simulink model "silnik elektryczny"  (R2025b)
settings: Solver=ode4  StartTime=0.0  StopTime=5  FixedStep=0.001  RelTol=1e-3
InitFcn:
  | Jzr = 0.027
  | Uamax = 220
  | Ra = 0.8
  | La = 0.1
  | Rf = 0.65
  | Lf = 0.1
  | Mo = 50
  | fobc = 13
  | k = 0.05
libraries: slpidlib x1, simulink x1
settings Model: Creator=maciuś  LastModifiedBy=maciuś

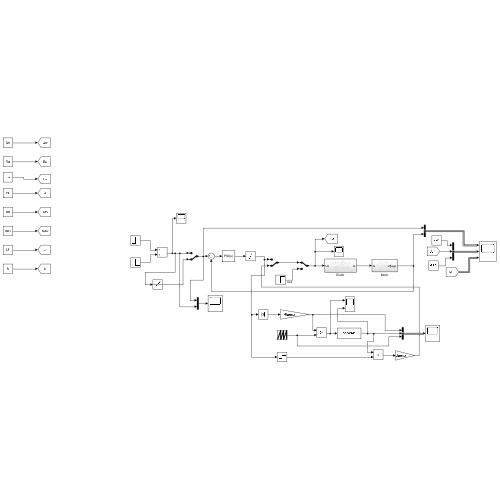
[thumbnail: Simulink's stored preview of the top-level diagram]
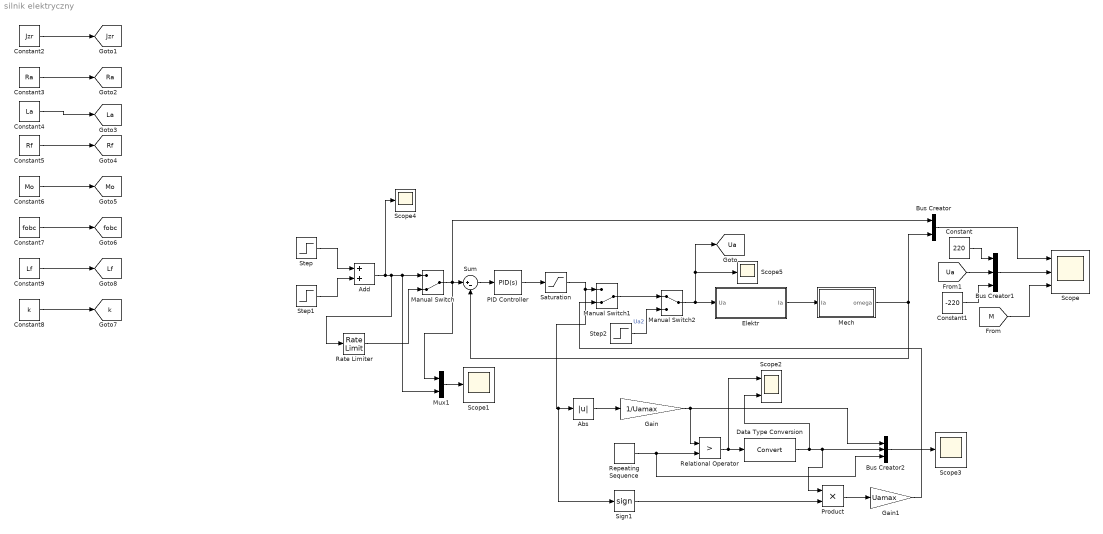
== system silnik elektryczny ==
  Abs : Abs  SaturateOnIntegerOverflow=off
  Add : Sum
  Bus Creator : BusCreator  Inputs=2
  Bus Creator1 : BusCreator  Inputs=3
  Bus Creator2 : BusCreator  Inputs=3
  Constant : Constant  Value=220
  Constant1 : Constant  Value=-220
  Constant2 : Constant  Value=Jzr
  Constant3 : Constant  Value=Ra
  Constant4 : Constant  Value=La
  Constant5 : Constant  Value=Rf
  Constant6 : Constant  Value=Mo
  Constant7 : Constant  Value=fobc
  Constant8 : Constant  Value=k
  Constant9 : Constant  Value=Lf
  Data Type Conversion : DataTypeConversion  SaturateOnIntegerOverflow=off  RndMeth=Floor
  Elektr : Subsystem
  Gain : Gain  Gain=1/Uamax
  Gain1 : Gain  Gain=Uamax
  Manual Switch : ManualSwitch  CurrentSetting=0
  Manual Switch1 : ManualSwitch  CurrentSetting=0
  Manual Switch2 : ManualSwitch
  Mech : Subsystem
  Mux1 : Mux  Inputs=2
  PID Controller : slpidlib/PID Controller  Controller=PID  Form=Ideal  TimeDomain=Continuous-time  UseExternalTs=off  SampleTime=-1  IntegratorMethod=Forward Euler  FilterMethod=Forward Euler  ControllerParametersSource=internal  P=8  I=5  UseKiTs=off  D=0.07  UseExternalDerivativeSource=off  N=100  UseFilter=on  TunerSelectOption=Transfer Function Based (PID Tuner App)  InitialConditionSource=internal  InitialConditionForIntegrator=0  InitialConditionForFilter=0  DifferentiatorICPrevScaledInput=0  ExternalReset=none  TrackingMode=off  Kt=1  LimitOutput=off  SatLimitsSource=internal  UpperSaturationLimit=inf  LowerSaturationLimit=-inf  LinearizeAsGain=on  AntiWindupMode=none  Kb=1  LimitIntegrator=off  UpperIntegratorSaturationLimit=inf  LowerIntegratorSaturationLimit=-inf  POutMin=[]  POutMax=[]  IOutMin=[]  IOutMax=[]  DOutMin=[]  DOutMax=[]  NOutMin=[]  NOutMax=[]  SumOutMin=[]  SumOutMax=[]  SaturationOutMin=[]  SaturationOutMax=[]  PParamMin=[]  PParamMax=[]  IParamMin=[]  IParamMax=[]  DParamMin=[]  DParamMax=[]  NParamMin=[]  NParamMax=[]  KbParamMin=[]  KbParamMax=[]  KtParamMin=[]  KtParamMax=[]  KbOutMin=[]  KbOutMax=[]  KtOutMin=[]  KtOutMax=[]  IntegratorOutMin=[]  IntegratorOutMax=[]  FilterOutMin=[]  FilterOutMax=[]  SumI1OutMin=[]  SumI1OutMax=[]  SumI2OutMin=[]  SumI2OutMax=[]  SumI3OutMin=[]  SumI3OutMax=[]  SumI4OutMin=[]  SumI4OutMax=[]  SumDOutMin=[]  SumDOutMax=[]  DifferentiatorOutMin=[]  DifferentiatorOutMax=[]  FilterDiffOutCoefMin=[]  FilterDiffOutCoefMax=[]  ReciprocalOutMin=[]  ReciprocalOutMax=[]  SumDenOutMin=[]  SumDenOutMax=[]  SumNumOutMin=[]  SumNumOutMax=[]  DivideOutMin=[]  DivideOutMax=[]  UdiffTsProdOutMin=[]  UdiffTsProdOutMax=[]  NTsProdOutMin=[]  NTsProdOutMax=[]  UintegralTsProdOutMin=[]  UintegralTsProdOutMax=[]  UngainTsProdOutMin=[]  UngainTsProdOutMax=[]  ClampingZeroOutDataTypeStr=Inherit: Inherit via back propagation  ClampingZeroOutMin=[]  ClampingZeroOutMax=[]  FilterDenConstantOutDataTypeStr=Inherit: Inherit via back propagation  FilterDenConstantOutMin=[]  FilterDenConstantOutMax=[]  PCopyOutDataTypeStr=Inherit: Inherit via back propagation  PCopyOutMin=[]  PCopyOutMax=[]  NCopyOutDataTypeStr=Inherit: Inherit via back propagation  NCopyOutMin=[]  NCopyOutMax=[]  IntegratorContinuousStateAttributes=''  IntegratorStateMustResolveToSignalObject=off  IntegratorRTWStateStorageClass=Auto  FilterContinuousStateAttributes=''  FilterStateMustResolveToSignalObject=off  FilterRTWStateStorageClass=Auto  ParallelPVariant=Passthrough  IdealPVariant=InternalParameters  IVariant=InternalParameters  DVariant=InternalParameters  IntegratorVariant=Continuous  SatVariant=Disabled  AWVariant=Passthrough  PCopyVariant=Disabled  TRVariant=Disabled  FdbkBlocksVariant=Forward  IdealPFdbkVariant=Disabled  SatFdbkVariant=Disabled  DerivativeFilterVariant=ContFilter  NVariant=InternalParameters  NCopyVariant=Disabled  FilterICVariant=InternalICsFilter  IntegratorICVariant=InternalICs  ExternalResetVariant=Disabled  TRSumVariant=Passthrough  SumFdbkVariant=Disabled  SumVariant=Sum_PID  TsampFilterVariant=InternalTs  TsampNgainVariant=Passthrough  TsampIntegralVariant=Disabled_SignalSpec  ExternalSaturationOutDataTypeStr=Inherit: Same as second input  DerivativeSourceVariant=ErrorSignal  PreIntVariant=InternalPreInt
  Product : Product
  Rate Limiter : RateLimiter  RisingSlewLimit=1000  FallingSlewLimit=-1000  SampleTimeMode=inherited
  Relational Operator : RelationalOperator  Operator=>  OutDataTypeStr=boolean  RndMeth=Simplest  InputSameDT=off
  Repeating Sequence : simulink/Sources/Repeating Sequence  rep_seq_t=[0 0.01]  rep_seq_y=[0 1]
  Saturation : Saturate  UpperLimit=220  LowerLimit=-220
  Scope : Scope  NumInputPorts=3
      settings: ActiveDisplayYMinimum=-62.522277874380592  ActiveDisplayYMaximum=126.43995774320904
  Scope{1,3..5} (4 alike) : Scope
      Scope1 settings: ActiveDisplayYMinimum=-28.272180553338188  ActiveDisplayYMaximum=212.0022706755459  DataLoggingVariableName=ScopeData3
      Scope3 settings: ActiveDisplayYMinimum=-0.12499999999999997  ActiveDisplayYMaximum=1.125  DataLoggingVariableName=ScopeData6
      Scope4 settings: ActiveDisplayYMinimum=-261.08167026296894  ActiveDisplayYMaximum=377.87326598282397  DataLoggingVariableName=ScopeData7
      Scope5 settings: ActiveDisplayYMinimum=-1  ActiveDisplayYMaximum=1  DataLoggingVariableName=ScopeData8
  Scope2 : Scope  NumInputPorts=2
      settings: ActiveDisplayYMinimum=-0.12499999999999997  ActiveDisplayYMaximum=1.125  DataLoggingVariableName=ScopeData5
  Sign1 : Signum
  Step : Step  After=4*13*2  SampleTime=0
  Step1 : Step  Time=2  After=-4*13  SampleTime=0
  Step2 : Step  After=Uamax  SampleTime=0
  Sum : Sum  Inputs=|+-
  tag scope: Jzr=global, La=global, Lf=global, Mo=global, Ra=global, Rf=global, Ua=global, fobc=global, k=global
  wires:
  Step/1 -> Add/1
  Step1/1 -> Add/2
  Add/1 -> Scope4/1, Rate Limiter/1, Mux1/2, Manual Switch/1
  Rate Limiter/1 -> Manual Switch/2
  Manual Switch/1 -> Sum/1, Bus Creator/1, Mux1/1
  Mux1/1 -> Scope1/1
  Sum/1 -> PID Controller/1
  PID Controller/1 -> Saturation/1
  Saturation/1 -> Sign1/1, Abs/1, Manual Switch1/1
  Manual Switch1/1 -> Manual Switch2/1
  Step2/1 -> Manual Switch2/2  "Ua2"
  Manual Switch2/1 -> Scope5/1, [Ua], Elektr/1(Ua)
  Elektr/1(Ia) -> Mech/1(Ia)
  Mech/1(omega) -> Sum/2, Bus Creator/2
  Bus Creator/1 -> Scope/1
  Bus Creator1/1 -> Scope/2
  [M] -> Scope/3
  [Ua] -> Bus Creator1/2
  Constant/1 -> Bus Creator1/1
  Constant1/1 -> Bus Creator1/3
  Abs/1 -> Gain/1
  Repeating Sequence/1 -> Bus Creator2/3, Relational Operator/2
  Relational Operator/1 -> Scope2/1, Data Type Conversion/1
  Gain/1 -> Bus Creator2/1, Relational Operator/1
  Bus Creator2/1 -> Scope3/1
  Gain1/1 -> Manual Switch1/2
  Product/1 -> Gain1/1
  Data Type Conversion/1 -> Scope2/2, Bus Creator2/2, Product/1
  Sign1/1 -> Product/2
  Constant2/1 -> [Jzr]
  Constant3/1 -> [Ra]
  Constant4/1 -> [La]
  Constant5/1 -> [Rf]
  Constant7/1 -> [fobc]
  Constant6/1 -> [Mo]
  Constant8/1 -> [k]
  Constant9/1 -> [Lf]

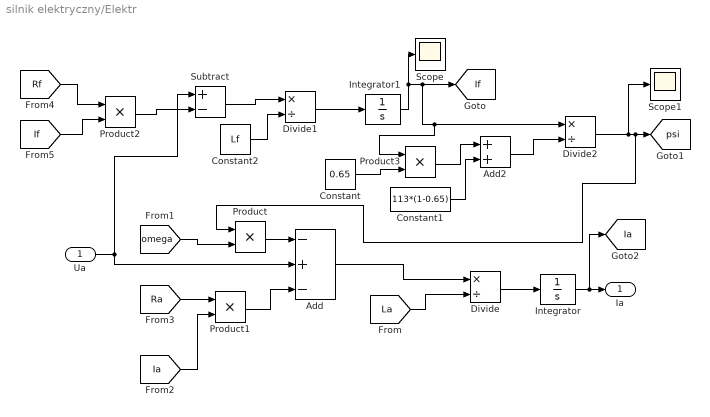
== system silnik elektryczny/Elektr ==
  Ua : Inport
  Add : Sum  Inputs=-+-
  Add2 : Sum
  Constant : Constant  Value=0.65
  Constant1 : Constant  Value=113*(1-0.65)
  Constant2 : Constant  Value=Lf
  Divide : Product  Inputs=*/
  Divide1 : Product  Inputs=*/
  Divide2 : Product  Inputs=*/
  Integrator : Integrator
  Integrator1 : Integrator
  Product{,1..3} (4 alike) : Product
  Scope : Scope
      settings: ActiveDisplayYMinimum=-56.7709575706929  ActiveDisplayYMaximum=445.30478054366728
  Scope1 : Scope
      settings: ActiveDisplayYMinimum=-3.1126452274013121  ActiveDisplayYMaximum=1.7057123763413438  DataLoggingVariableName=ScopeData2
  Subtract : Sum  Inputs=+-
  Ia : Outport
  tag scope: Ia=global, If=global, psi=global
  wires:
  Integrator/1 -> [Ia], Ia/1
  Divide/1 -> Integrator/1
  [La] -> Divide/2
  Add/1 -> Divide/1
  Product1/1 -> Add/3
  [Ia] -> Product1/2
  [Ra] -> Product1/1
  [Rf] -> Product2/1
  [If] -> Product2/2
  Product2/1 -> Subtract/2
  Ua/1 -> Subtract/1, Add/2
  Subtract/1 -> Divide1/1
  Divide1/1 -> Integrator1/1
  Integrator1/1 -> Product3/1, Divide2/1, [If], Scope/1
  Add2/1 -> Divide2/2
  Product3/1 -> Add2/1
  Constant/1 -> Product3/2
  Constant1/1 -> Add2/2
  Constant2/1 -> Divide1/2
  [omega] -> Product/2
  Product/1 -> Add/1
  Divide2/1 -> Scope1/1, Product/1, [psi]

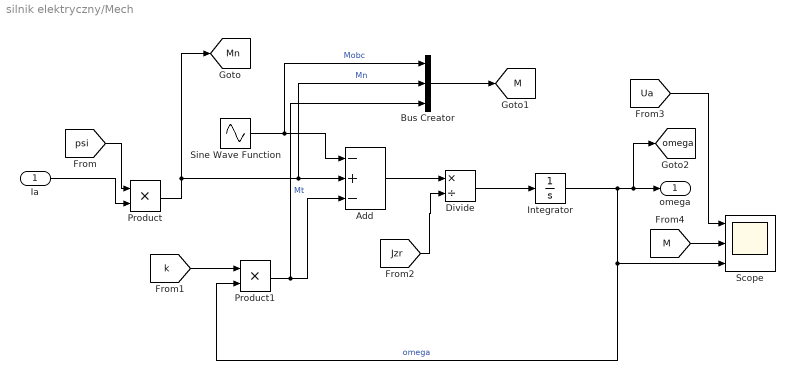
== system silnik elektryczny/Mech ==
  Ia : Inport
  Add : Sum  Inputs=-+-
  Bus Creator : BusCreator  Inputs=3
  Divide : Product  Inputs=*/
  Integrator : Integrator
  Product : Product
  Product1 : Product
  Scope : Scope  NumInputPorts=3
      settings: ActiveDisplayYMinimum=-27.499999999999993  ActiveDisplayYMaximum=247.5  DataLoggingVariableName=ScopeData4
  Sine Wave Function : Sin  Amplitude=0.25*Mo  Bias=Mo  Frequency=2*pi*fobc  SampleTime=0.001
  omega : Outport
  tag scope: M=global, Mn=global, omega=global
  wires:
  Ia/1 -> Product/2
  [psi] -> Product/1
  Product/1 -> [Mn], Bus Creator/2, Add/2  "Mn"
  Sine Wave Function/1 -> Bus Creator/1, Add/1  "Mobc"
  Bus Creator/1 -> [M]
  [k] -> Product1/1
  Product1/1 -> Bus Creator/3, Add/3  "Mt"
  Add/1 -> Divide/1
  [Jzr] -> Divide/2
  Divide/1 -> Integrator/1
  Integrator/1 -> Scope/3, Product1/2, [omega], omega/1  "omega"
  [Ua] -> Scope/1
  [M] -> Scope/2
